simulink model "Sim_LQR_Skid_Steer_rover"  (R2014a)
settings: Solver=ode4  StartTime=0.0  StopTime=100  FixedStep=0.06  RelTol=1e-3
values from neighbouring files (symbols this model uses):
  A = [-inv(MP_bar)*CP_bar zeros(2,1) inv(MP_bar)*B_km;     -r/(Yl+Yr) r/(Yl+Yr) zeros(1,3);     -Kbl*N/La 0 0 -Ra/La 0;     0 -Kbr*N/La 0 0 -Ra/La]    [Diseno_controlador_LQR_skid_steer.m]    (also in MPC_Rover_settings.m; S_Rover_skid_steer.m = [-inv(M_b*P)*C_b*P zeros(2,1) inv(M_b*P)*B_b*Km;     -r/(Yl+)
  B = Kpwm/La*[zeros(3,2);eye(2)]    [Diseno_controlador_LQR_skid_steer.m]    (also in MPC_Rover_settings.m; S_Rover_skid_steer.m = [zeros(3,2);Kpwm/La 0;0 Kpwm/La])
  C = [0 0 1 0 0;0.5*0.2 0.5*0.2 0 0 0]    [Diseno_controlador_LQR_skid_steer.m]    (also in MPC_Rover_settings.m)
  K = Ka(:,1:5)    [Diseno_controlador_LQR_skid_steer.m]
  Ki = Ka(:,6:7)    [Diseno_controlador_LQR_skid_steer.m]
  T = 60e-3    (= 0.06)    [Diseno_controlador_LQR_skid_steer.m]
undefined symbols (not defined in the file or in its folder): sigbuilder_block
settings Model: Creator=obarrero  LastModifiedBy=obarrero
settings DataIOCC: SignalLoggingSaveFormat=ModelDataLogs
settings DebuggingCC: MultiTaskDSMMsg=warning  MultiTaskCondExecSysMsg=none  StrictBusMsg=ErrorOnBusTreatedAsVector
settings RTWCC: IncludeERTFirstTime=on

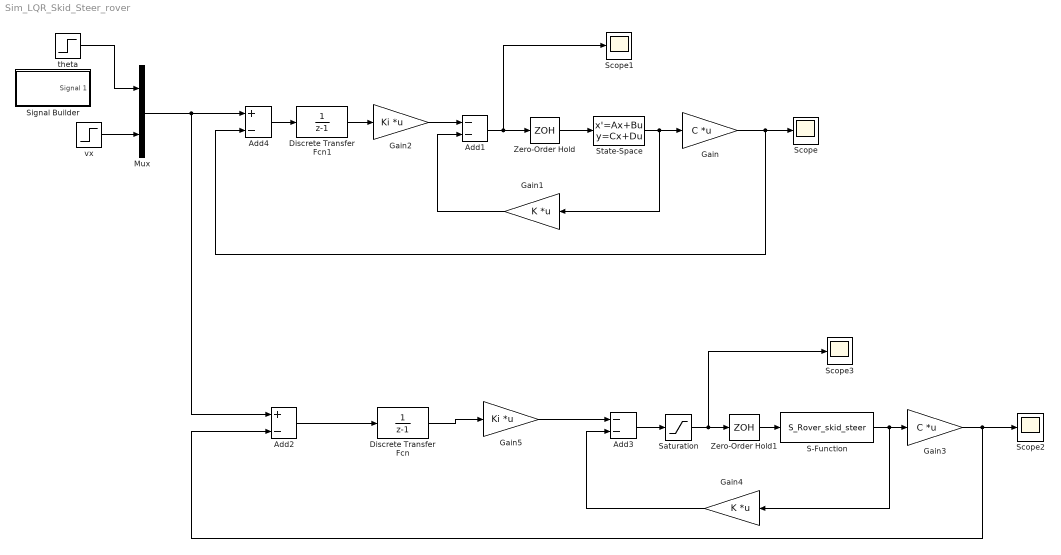
== system Sim_LQR_Skid_Steer_rover ==
  Add1 : Sum  Inputs=--
  Add2 : Sum  Inputs=+-
  Add3 : Sum  Inputs=--
  Add4 : Sum  Inputs=+-
  Discrete Transfer Fcn : DiscreteTransferFcn  Denominator=[1 -1]  SampleTime=T
  Discrete Transfer Fcn1 : DiscreteTransferFcn  Denominator=[1 -1]  SampleTime=T
  Gain : Gain  Gain=C  Multiplication=Matrix(K*u) (u vector)  SampleTime=T
  Gain1 : Gain  Gain=K  Multiplication=Matrix(K*u) (u vector)  SampleTime=T
  Gain2 : Gain  Gain=Ki  Multiplication=Matrix(K*u) (u vector)  SampleTime=T
  Gain3 : Gain  Gain=C  Multiplication=Matrix(K*u) (u vector)  SampleTime=T
  Gain4 : Gain  Gain=K  Multiplication=Matrix(K*u) (u vector)  SampleTime=T
  Gain5 : Gain  Gain=Ki  Multiplication=Matrix(K*u) (u vector)  SampleTime=T
  Mux : Mux  Inputs=2
  S-Function : S-Function  FunctionName=S_Rover_skid_steer  EnableBusSupport=off
  Saturation : Saturate  UpperLimit=100  LowerLimit=-100
  Scope{,1..3} (4 alike) : Scope
      Scope settings: YMin=0  YMax=0.11
      Scope2 settings: YMin=-0.5  YMax=7  SaveName=ScopeData2
      Scope3 settings: YMin=-60  YMax=80  SaveName=ScopeData3
  Signal Builder : Subsystem  Tag=STV Subsys  LoadFcn=sigbuilder_block('load');  StartFcn=sigbuilder_block('start');  StopFcn=sigbuilder_block('stop');  ClipboardFcn=sigbuilder_block('clipboard');  mask(Sigbuilder block){}
      mask help: Simulink:masks:SigbuilderBlock_MD
      mask init:
      | if ~strcmp(get_param(bdroot(gcbh),'SimulationStatus'),'stopped') tuvar = sigbuilder_block('maskInit'); end
      settings: CopyFcn=sigbuilder_block('copy');  DeleteFcn=sigbuilder_block('delete');  ModelCloseFcn=sigbuilder_block('modelClose');  PreSaveFcn=sigbuilder_block('preSave');  PauseFcn=sigbuilder_block('pause');  ContinueFcn=sigbuilder_block('continue');  NameChangeFcn=sigbuilder_block('namechange');  OpenFcn=sigbuilder_block('open',[439.5 117 550.5 395.25 ]);  CloseFcn=sigbuilder_block('close');
      mask Display: plot(0, 0, 100, 100,[2, 2, 32, 32, 2], [68, 8, 8, 68, 68],[32, 2], [38, 38], [32, 19, 2],[53, 60, 44], [32, 17, 17, 2],[16, 16, 31, 31]);txt = getActiveGroup(gcbh);text(2, 100, txt,'verticalAlignment', 'top');
  State-Space : StateSpace  A=A  B=B  C=eye(5)  D=zeros(5,2)  X0=[0 0 0.92 0 0]
  Zero-Order Hold : ZeroOrderHold  SampleTime=T
  Zero-Order Hold1 : ZeroOrderHold  SampleTime=T
  theta : Step  Time=0  After=pi/4  SampleTime=0
  vx : Step  Time=0  SampleTime=0
  wires:
  Zero-Order Hold/1 -> State-Space/1
  State-Space/1 -> Gain1/1, Gain/1
  Gain/1 -> Add4/2, Scope/1
  Add1/1 -> Scope1/1, Zero-Order Hold/1
  Gain1/1 -> Add1/2
  Gain2/1 -> Add1/1
  vx/1 -> Mux/2
  Zero-Order Hold1/1 -> S-Function/1
  Add3/1 -> Saturation/1
  Gain4/1 -> Add3/2
  S-Function/1 -> Gain4/1, Gain3/1
  Saturation/1 -> Scope3/1, Zero-Order Hold1/1
  Mux/1 -> Add2/1, Add4/1
  theta/1 -> Mux/1
  Gain3/1 -> Add2/2, Scope2/1
  Add2/1 -> Discrete Transfer Fcn/1
  Discrete Transfer Fcn/1 -> Gain5/1
  Gain5/1 -> Add3/1
  Add4/1 -> Discrete Transfer Fcn1/1
  Discrete Transfer Fcn1/1 -> Gain2/1

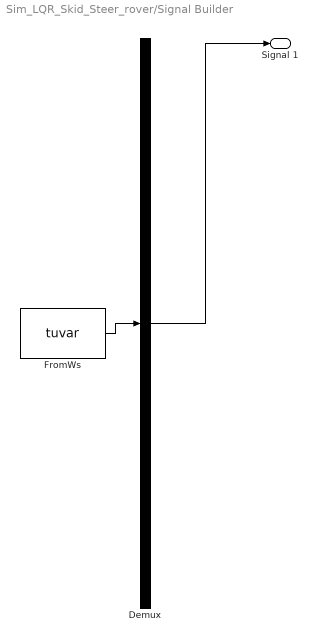
== system Sim_LQR_Skid_Steer_rover/Signal Builder ==
  Demux : Demux  Tag=STV Demux  Outputs=1
  FromWs : FromWorkspace  Tag=STV FromWs  VariableName=tuvar  SampleTime=0
      SigBuilderData=|
      | common.afterFinalStr = 'Extrapolate'
      | common.sampleTime = 0
      | dataSet.timeRange = [0 100]
      | dataSet.name = 'Group 1'
      | sbobj.Groups.Name = 'Group 1'
      | sbobj.Groups.Signals.Name = 'Signal 1'
      | sbobj.Groups.Signals.XData = [0 10 15 25 30 40 45 55 60 100]
      | sbobj.Groups.Signals.YData = [0 0 1.57079632679 1.58 3.14159265359 3.14159265359 4.71238898038 4.71238898038 6.28318530718 6.28318530718]
      | sbobj.Groups.TimeRange = [0 100]
  Signal 1 : Outport  Tag=STV Outport
  wires:
  Demux/1 -> Signal 1/1
  FromWs/1 -> Demux/1
